simulink model "lab5_Sim"  (R2017b)
settings: Solver=VariableStepAuto  StartTime=0.0  StopTime=10.0  RelTol=1e-3
InitFcn:
  | load speech_signal
  | Fs= 8000;
  | Ts= 1/Fs;
  | 
  | DPRAM1_size = 2048;
  | DPRAM1_address_size = log2(DPRAM1_size);
  | 
  | FFT_size = 1024;
  | FFT_size_half = FFT_size;
  | FFT_frame_shift = 256;
  | FFT_frame_shift_Nbits = log2(FFT_frame_shift);
  | 
  | SysRate_Upsample_Factor = 32;
libraries: hdlsllib x16, simulink x5, dspxfrm3 x2, dspsigops x1
settings Model: Creator=Ross_admin  LastModifiedBy=h92j874
settings OptimizationCC: BlockReduction=off  ConditionallyExecuteInputs=off  DefaultParameterBehavior=Inlined
settings DebuggingCC: AlgebraicLoopMsg=error
settings HardwareCC: ProdBitPerPointer=32  ProdBitPerSizeT=32  ProdBitPerPtrDiffT=32  ProdLargestAtomicFloat=None  ProdIntDivRoundTo=Undefined  ProdEndianess=Unspecified  ProdWordSize=32  ProdHWDeviceType=ASIC/FPGA->ASIC/FPGA  TargetBitPerPointer=64  TargetBitPerSizeT=64  TargetBitPerPtrDiffT=64  TargetLongLongMode=on  TargetIntDivRoundTo=Zero  TargetEndianess=LittleEndian  TargetWordSize=64  TargetHWDeviceType=Custom Processor->MATLAB Host Computer  ProdEqTarget=off
settings CodeAppCC: StateflowObjectComments=on

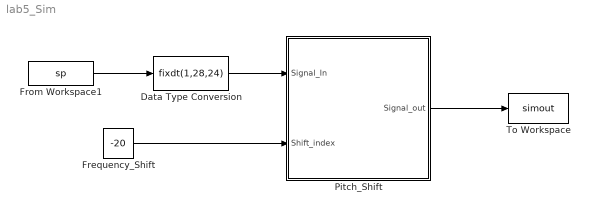
== system lab5_Sim ==
  Data Type Conversion : DataTypeConversion  OutDataTypeStr=fixdt(1,28,24)
  Frequency_Shift : Constant  Value=-20  OutDataTypeStr=int16
  From Workspace1 : FromWorkspace  VariableName=sp  SampleTime=0
  Pitch_Shift : Subsystem
  To Workspace : ToWorkspace  VariableName=simout  SampleTime=-1
  wires:
  Frequency_Shift/1 -> Pitch_Shift/2(Shift_index)
  Data Type Conversion/1 -> Pitch_Shift/1(Signal_In)
  From Workspace1/1 -> Data Type Conversion/1
  Pitch_Shift/1(Signal_out) -> To Workspace/1

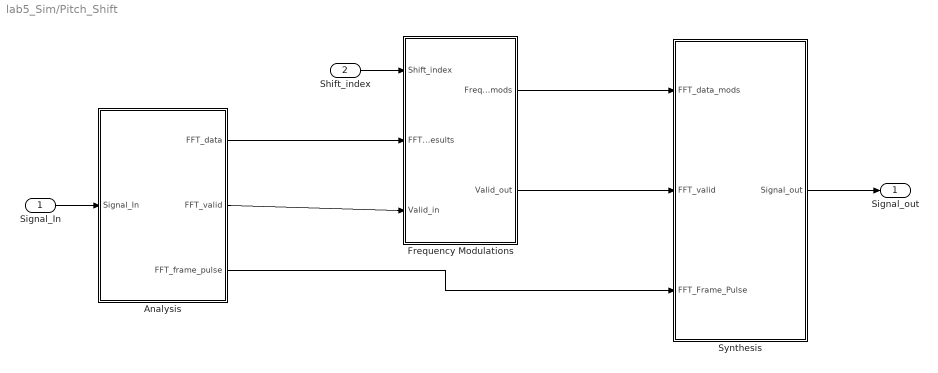
== system lab5_Sim/Pitch_Shift ==
  Signal_In : Inport
  Shift_index : Inport  Port=2
  Analysis : Subsystem
  Frequency Modulations : Subsystem
  Synthesis : Subsystem
  Signal_out : Outport
  wires:
  Signal_In/1 -> Analysis/1("Signal_In ")
  Analysis/1(FFT_data) -> Frequency Modulations/2(FFT_Results)
  Analysis/2(FFT_valid) -> Frequency Modulations/3(Valid_in)
  Shift_index/1 -> Frequency Modulations/1(Shift_index)
  Frequency Modulations/1(Frequency_mods) -> Synthesis/1(FFT_data_mods)
  Frequency Modulations/2(Valid_out) -> Synthesis/2(FFT_valid)
  Synthesis/1(Signal_out) -> Signal_out/1
  Analysis/3(FFT_frame_pulse) -> Synthesis/3(FFT_Frame_Pulse)

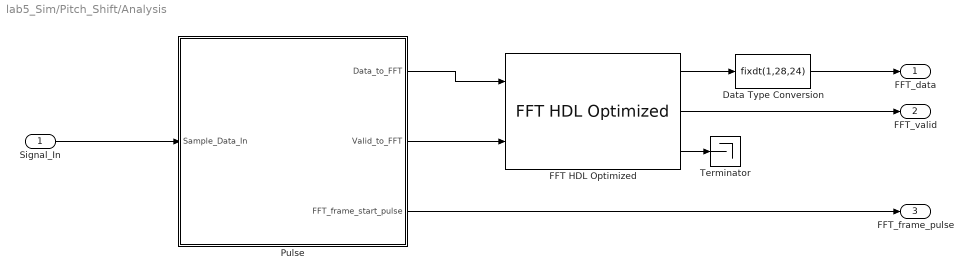
== system lab5_Sim/Pitch_Shift/Analysis ==
  "Signal_In " : Inport
  Data Type Conversion : DataTypeConversion  OutDataTypeStr=fixdt(1,28,24)
  FFT HDL Optimized : dspxfrm3/FFT HDL Optimized  FFTLength=1024  Architecture=Burst Radix 2  ComplexMultiplication=Use 4 multipliers and 2 adders  BitReversedOutput=off  BitReversedInput=off  Normalize=on  SimulateUsing=Code generation  RoundingMethod=Floor  ResetInputPort=off  StartOutputPort=off  EndOutputPort=off
      settings: SourceProductName=DSP System Toolbox  SourceProductBaseCode=DS
  "Pulse " : Subsystem
  Terminator : Terminator
  FFT_data : Outport
  FFT_valid : Outport  Port=2
  FFT_frame_pulse : Outport  Port=3
  wires:
  "Signal_In "/1 -> "Pulse "/1(Sample_Data_In)
  "Pulse "/3(FFT_frame_start_pulse) -> FFT_frame_pulse/1
  "Pulse "/2(Valid_to_FFT) -> FFT HDL Optimized/2
  FFT HDL Optimized/1 -> Data Type Conversion/1
  Data Type Conversion/1 -> FFT_data/1
  FFT HDL Optimized/2 -> FFT_valid/1
  FFT HDL Optimized/3 -> Terminator/1
  "Pulse "/1("Data_to_FFT ") -> FFT HDL Optimized/1

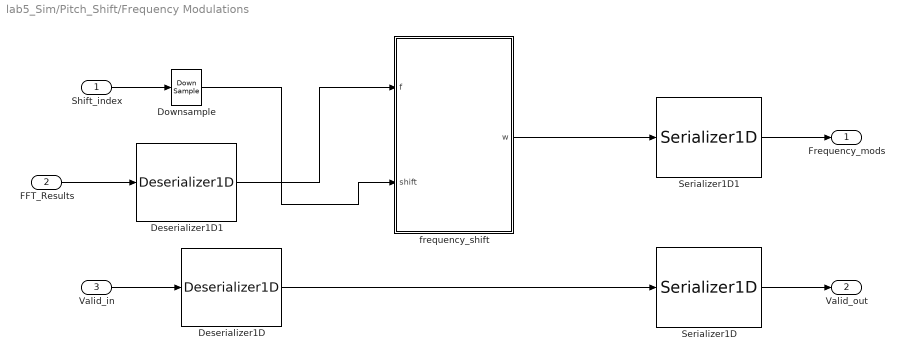
== system lab5_Sim/Pitch_Shift/Frequency Modulations ==
  Shift_index : Inport
  FFT_Results : Inport  Port=2
  Valid_in : Inport  Port=3
  Deserializer1D : hdlsllib/HDL Operations/Deserializer1D  Ratio=1024  IdleCycles=0  InitialCondition=0  startIn=off  validIn=off  validOut=off  inputDataDimensions=-1  inputSampleTime=-1  inputSignalType=auto
      settings: SourceProductName=HDL Coder  SourceProductBaseCode=HD
  Deserializer1D1 : hdlsllib/HDL Operations/Deserializer1D  Ratio=1024  IdleCycles=0  InitialCondition=0  startIn=off  validIn=off  validOut=off  inputDataDimensions=-1  inputSampleTime=-1  inputSignalType=auto
      settings: SourceProductName=HDL Coder  SourceProductBaseCode=HD
  Downsample : DownSample  N=FFT_size  RateOptions=Allow multirate processing
  Serializer1D : hdlsllib/HDL Operations/Serializer1D  Ratio=1024  IdleCycles=0  validIn=off  startOut=off  validOut=off  inputDataDimensions=-1  inputSampleTime=-1  inputSignalType=auto
      settings: SourceProductName=HDL Coder  SourceProductBaseCode=HD
  Serializer1D1 : hdlsllib/HDL Operations/Serializer1D  Ratio=1024  IdleCycles=0  validIn=off  startOut=off  validOut=off  inputDataDimensions=-1  inputSampleTime=-1  inputSignalType=auto
      settings: SourceProductName=HDL Coder  SourceProductBaseCode=HD
  "frequency_shift " : MATLAB Function  TreatAsAtomicUnit=on
  Frequency_mods : Outport
  Valid_out : Outport  Port=2
  wires:
  Serializer1D1/1 -> Frequency_mods/1
  FFT_Results/1 -> Deserializer1D1/1
  Valid_in/1 -> Deserializer1D/1
  Shift_index/1 -> Downsample/1
  "frequency_shift "/1(w) -> Serializer1D1/1
  Serializer1D/1 -> Valid_out/1
  Downsample/1 -> "frequency_shift "/2(shift)
  Deserializer1D1/1 -> "frequency_shift "/1(f)
  Deserializer1D/1 -> Serializer1D/1

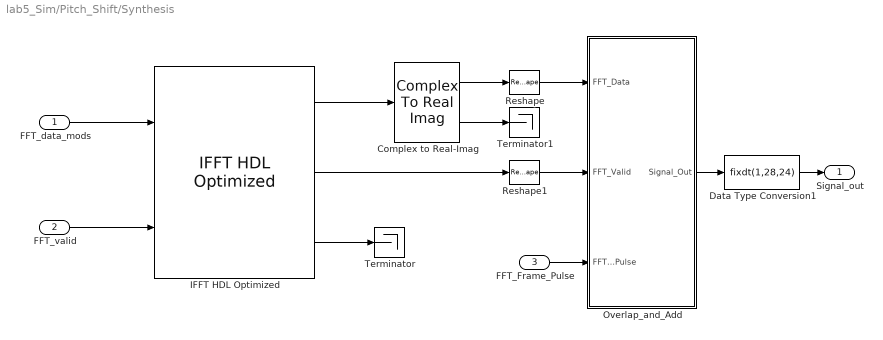
== system lab5_Sim/Pitch_Shift/Synthesis ==
  FFT_data_mods : Inport
  FFT_valid : Inport  Port=2
  FFT_Frame_Pulse : Inport  Port=3
  Complex to Real-Imag : ComplexToRealImag
  Data Type Conversion1 : DataTypeConversion  OutDataTypeStr=fixdt(1,28,24)
  IFFT HDL Optimized : dspxfrm3/IFFT HDL Optimized  FFTLength=1024  Architecture=Burst Radix 2  ComplexMultiplication=Use 4 multipliers and 2 adders  BitReversedOutput=off  BitReversedInput=off  Normalize=on  SimulateUsing=Code generation  RoundingMethod=Floor  ResetInputPort=off  StartOutputPort=off  EndOutputPort=off
      settings: SourceProductName=DSP System Toolbox  SourceProductBaseCode=DS
  Overlap_and_Add : Subsystem
  Reshape : Reshape
  Reshape1 : Reshape
  Terminator : Terminator
  Terminator1 : Terminator
  Signal_out : Outport
  wires:
  FFT_data_mods/1 -> IFFT HDL Optimized/1
  FFT_valid/1 -> IFFT HDL Optimized/2
  IFFT HDL Optimized/3 -> Terminator/1
  IFFT HDL Optimized/1 -> Complex to Real-Imag/1
  Complex to Real-Imag/1 -> Reshape/1
  Complex to Real-Imag/2 -> Terminator1/1
  IFFT HDL Optimized/2 -> Reshape1/1
  Reshape1/1 -> Overlap_and_Add/2(FFT_Valid)
  Reshape/1 -> Overlap_and_Add/1(FFT_Data)
  FFT_Frame_Pulse/1 -> Overlap_and_Add/3(FFT_Frame_Pulse)
  Data Type Conversion1/1 -> Signal_out/1
  Overlap_and_Add/1(Signal_Out) -> Data Type Conversion1/1

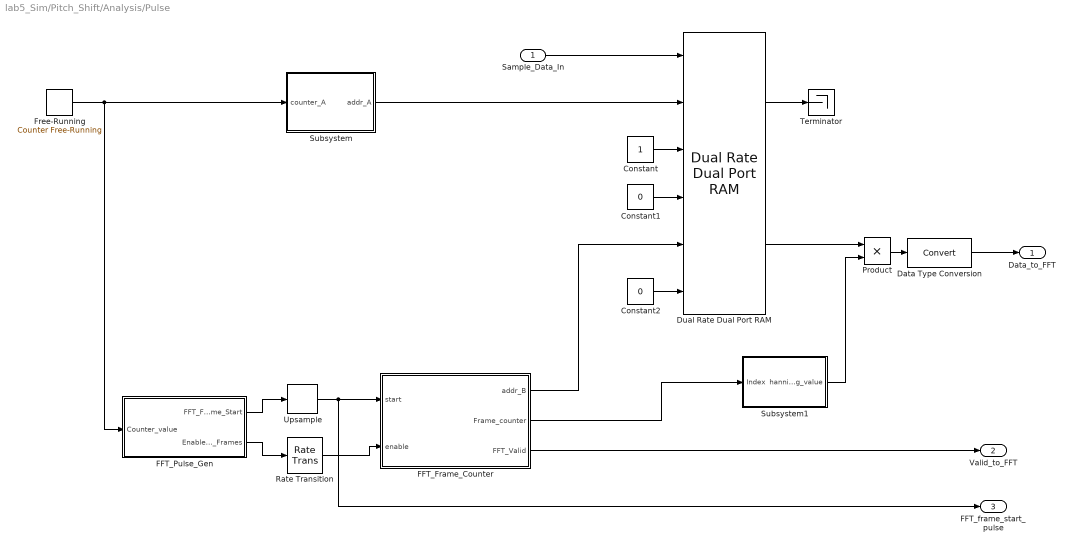
== system lab5_Sim/Pitch_Shift/Analysis/Pulse  ==
  Sample_Data_In : Inport
  Constant : Constant  OutDataTypeStr=boolean
  Constant1 : Constant  Value=0  OutDataTypeStr=fixdt(1,28,24)
  Constant2 : Constant  Value=0  OutDataTypeStr=boolean
  Data Type Conversion : DataTypeConversion
  Dual Rate Dual Port RAM : hdlsllib/HDL RAMs/Dual Rate Dual Port RAM  ram_size=DPRAM1_address_size
      settings: SourceProductName=HDL Coder  SourceProductBaseCode=HD
  FFT_Frame_Counter : Subsystem
  FFT_Pulse_Gen : Subsystem
  Free-Running : simulink/Sources/Counter Free-Running  NumBits=DPRAM1_address_size  tsamp=Ts
  Product : Product
  Rate Transition : RateTransition
  Subsystem : Subsystem
  Subsystem1 : Subsystem
  Terminator : Terminator
  Upsample : dspsigops/Upsample  N=SysRate_Upsample_Factor  phase=0  RateOptions=Allow multirate processing  ic=0  mode=Unused parameter value
  "Data_to_FFT " : Outport
  Valid_to_FFT : Outport  Port=2
  FFT_frame_start_pulse : Outport  Port=3
  wires:
  FFT_Pulse_Gen/2(Enable_FFT_Frames) -> Rate Transition/1
  Subsystem1/1(hanning_value) -> Product/2
  Subsystem/1(addr_A) -> Dual Rate Dual Port RAM/2
  FFT_Frame_Counter/1(addr_B) -> Dual Rate Dual Port RAM/5
  Dual Rate Dual Port RAM/2 -> Product/1
  FFT_Frame_Counter/3("FFT_Valid ") -> Valid_to_FFT/1
  Upsample/1 -> FFT_frame_start_pulse/1, FFT_Frame_Counter/1("start ")
  Rate Transition/1 -> FFT_Frame_Counter/2("enable ")
  FFT_Frame_Counter/2("Frame_counter ") -> Subsystem1/1(Index)
  FFT_Pulse_Gen/1("FFT_Frame_Start ") -> Upsample/1
  Free-Running/1 -> Subsystem/1("counter_A "), FFT_Pulse_Gen/1("Counter_value ")
  Constant2/1 -> Dual Rate Dual Port RAM/6
  Constant/1 -> Dual Rate Dual Port RAM/3
  Sample_Data_In/1 -> Dual Rate Dual Port RAM/1
  Constant1/1 -> Dual Rate Dual Port RAM/4
  Product/1 -> Data Type Conversion/1
  Data Type Conversion/1 -> "Data_to_FFT "/1
  Dual Rate Dual Port RAM/1 -> Terminator/1

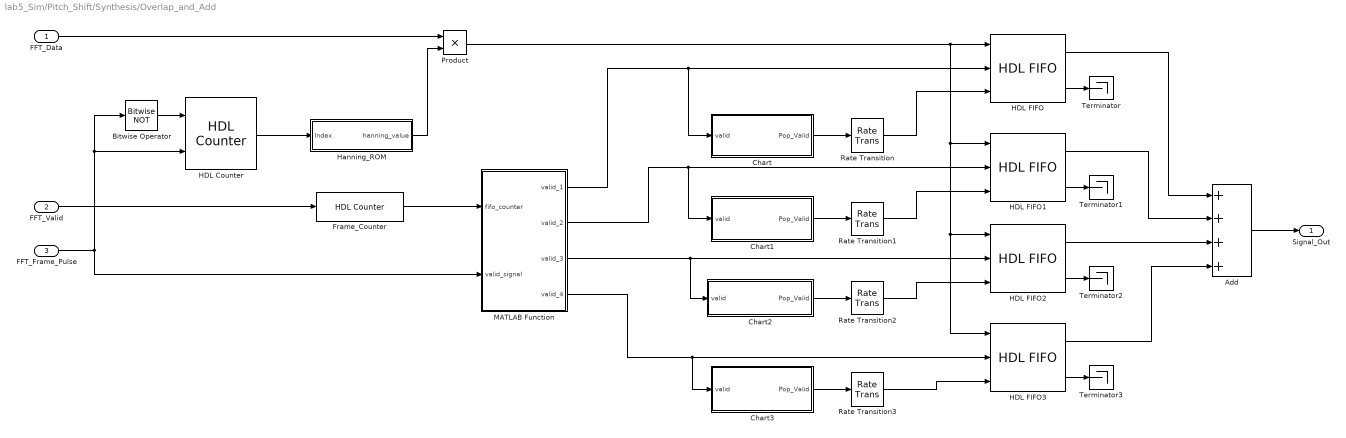
== system lab5_Sim/Pitch_Shift/Synthesis/Overlap_and_Add ==
  FFT_Data : Inport
  FFT_Valid : Inport  Port=2
  FFT_Frame_Pulse : Inport  Port=3
  Add : Sum  Inputs=4
  Bitwise Operator : simulink/Logic and Bit Operations/Bitwise Operator  logicop=NOT  UseBitMask=off  BitMask=bin2dec('11011001')  BitMaskRealWorld=Stored Integer
  Chart : Stateflow chart  TreatAsAtomicUnit=on
  Chart1 : Stateflow chart  TreatAsAtomicUnit=on
  Chart2 : Stateflow chart  TreatAsAtomicUnit=on
  Chart3 : Stateflow chart  TreatAsAtomicUnit=on
  Frame_Counter : hdlsllib/Sources/HDL Counter  CountType=Free running  CountInit=2  CountStep=1  CountMax=3  CountFromType=Initial value  CountFrom=2  CountResetPort=off  CountLoadPort=off  CountEnbPort=on  CountDirPort=off  CountDataType=Unsigned  CountWordLen=2  CountFracLen=0  CountSampTime=1
      settings: SourceProductBaseCode=HD
  HDL Counter : hdlsllib/Sources/HDL Counter  CountType=Count limited  CountInit=0  CountStep=1  CountMax=FFT_size  CountFromType=Initial value  CountFrom=0  CountResetPort=on  CountLoadPort=off  CountEnbPort=on  CountDirPort=off  CountDataType=Unsigned  CountWordLen=DPRAM1_address_size  CountFracLen=0  CountSampTime=1
      settings: SourceProductBaseCode=HD
  HDL FIFO{,1..3} (4 alike) : hdlsllib/HDL RAMs/HDL FIFO  fifo_size=FFT_size  ratio=SysRate_Upsample_Factor  push_msg=Warning  pop_msg=Warning  show_empty=off  show_full=on  show_num=off
      settings: SourceProductName=HDL Coder  SourceProductBaseCode=HD
  Hanning_ROM : Subsystem
  MATLAB Function : MATLAB Function  TreatAsAtomicUnit=on
  Product : Product
  Rate Transition{,1..3} (4 alike) : RateTransition  OutPortSampleTimeOpt=Multiple of input port sample time  OutPortSampleTimeMultiple=SysRate_Upsample_Factor  OutPortSampleTime=SysRate_Upsample_Factor
  Terminator{,1..3} (4 alike) : Terminator
  Signal_Out : Outport
  wires:
  Bitwise Operator/1 -> HDL Counter/1
  FFT_Frame_Pulse/1 -> MATLAB Function/2(valid_signal), HDL Counter/2, Bitwise Operator/1
  FFT_Data/1 -> Product/1
  HDL Counter/1 -> Hanning_ROM/1(Index)
  Hanning_ROM/1(hanning_value) -> Product/2
  FFT_Valid/1 -> Frame_Counter/1
  Frame_Counter/1 -> MATLAB Function/1(fifo_counter)
  Chart3/1(Pop_Valid) -> Rate Transition3/1
  Add/1 -> Signal_Out/1
  Product/1 -> HDL FIFO1/1, HDL FIFO3/1, HDL FIFO2/1, HDL FIFO/1
  MATLAB Function/2(valid_2) -> Chart1/1(valid), HDL FIFO1/2
  MATLAB Function/3(valid_3) -> Chart2/1(valid), HDL FIFO2/2
  MATLAB Function/4(valid_4) -> Chart3/1(valid), HDL FIFO3/2
  MATLAB Function/1(valid_1) -> Chart/1(valid), HDL FIFO/2
  Rate Transition3/1 -> HDL FIFO3/3
  Rate Transition2/1 -> HDL FIFO2/3
  Rate Transition1/1 -> HDL FIFO1/3
  Rate Transition/1 -> HDL FIFO/3
  HDL FIFO/1 -> Add/1
  HDL FIFO1/1 -> Add/2
  HDL FIFO2/1 -> Add/3
  HDL FIFO3/1 -> Add/4
  HDL FIFO1/2 -> Terminator1/1
  HDL FIFO2/2 -> Terminator2/1
  HDL FIFO3/2 -> Terminator3/1
  HDL FIFO/2 -> Terminator/1
  Chart1/1(Pop_Valid) -> Rate Transition1/1
  Chart/1(Pop_Valid) -> Rate Transition/1
  Chart2/1(Pop_Valid) -> Rate Transition2/1

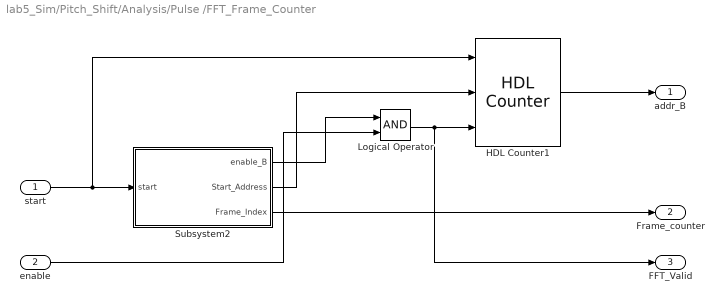
== system lab5_Sim/Pitch_Shift/Analysis/Pulse /FFT_Frame_Counter ==
  "start " : Inport
  "enable " : Inport  Port=2
  HDL Counter1 : hdlsllib/Sources/HDL Counter  CountType=Count limited  CountInit=DPRAM1_size-10  CountStep=1  CountMax=1024  CountFromType=Specify  CountFrom=DPRAM1_size-10  CountResetPort=off  CountLoadPort=on  CountEnbPort=on  CountDirPort=off  CountDataType=Unsigned  CountWordLen=DPRAM1_address_size  CountFracLen=0  CountSampTime=1
      settings: SourceProductBaseCode=HD
  Logical Operator : Logic  AllPortsSameDT=off  OutDataTypeStr=boolean
  Subsystem2 : Subsystem
  addr_B : Outport
  "Frame_counter " : Outport  Port=2
  "FFT_Valid " : Outport  Port=3
  wires:
  Subsystem2/1(enable_B) -> Logical Operator/1
  "start "/1 -> HDL Counter1/1, Subsystem2/1("start ")
  HDL Counter1/1 -> addr_B/1
  Logical Operator/1 -> "FFT_Valid "/1, HDL Counter1/3
  Subsystem2/2(Start_Address) -> HDL Counter1/2
  Subsystem2/3("Frame_Index ") -> "Frame_counter "/1
  "enable "/1 -> Logical Operator/2

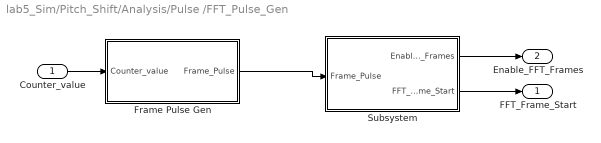
== system lab5_Sim/Pitch_Shift/Analysis/Pulse /FFT_Pulse_Gen ==
  "Counter_value " : Inport
  "Frame Pulse Gen " : Subsystem
  Subsystem : Subsystem
  "FFT_Frame_Start " : Outport
  Enable_FFT_Frames : Outport  Port=2
  wires:
  "Frame Pulse Gen "/1("Frame_Pulse ") -> Subsystem/1("Frame_Pulse ")
  Subsystem/1(Enable_FFT_Frames) -> Enable_FFT_Frames/1
  Subsystem/2("FFT_Frame_Start ") -> "FFT_Frame_Start "/1
  "Counter_value "/1 -> "Frame Pulse Gen "/1("Counter_value ")

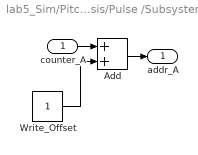
== system lab5_Sim/Pitch_Shift/Analysis/Pulse /Subsystem ==
  "counter_A " : Inport
  Add : Sum  AccumDataTypeStr=fixdt(0,11,0)
  "Write_Offset " : Constant  OutDataTypeStr=fixdt(0,11,0)
  addr_A : Outport
  wires:
  "Write_Offset "/1 -> Add/2
  "counter_A "/1 -> Add/1
  Add/1 -> addr_A/1

== system lab5_Sim/Pitch_Shift/Analysis/Pulse /Subsystem1 ==
  Index : Inport
  1-D Lookup Table1 : Lookup_n-D  NumberOfTableDimensions=1  LookupTableObject=''  BreakpointsForDimension1=[0:FFT_size]  BreakpointsForDimension1FirstPoint=10  BreakpointsForDimension2FirstPoint=10  BreakpointsForDimension1Spacing=12  BreakpointsForDimension2Spacing=12  IndexSearchMethod=Evenly spaced points  Table=hanning(FFT_size+1)  InterpMethod=Flat  DiagnosticForOutOfRangeInput=Error  OutDataTypeStr=fixdt(1,16,14)  RndMeth=Simplest  InputSameDT=on
  Unit Delay : UnitDelay  SampleTime=-1
  hanning_value : Outport
  wires:
  1-D Lookup Table1/1 -> Unit Delay/1
  Unit Delay/1 -> hanning_value/1
  Index/1 -> 1-D Lookup Table1/1

== system lab5_Sim/Pitch_Shift/Synthesis/Overlap_and_Add/Hanning_ROM ==
  Index : Inport
  1-D Lookup Table : Lookup_n-D  NumberOfTableDimensions=1  LookupTableObject=''  BreakpointsForDimension1=[0:FFT_size]  BreakpointsForDimension1FirstPoint=10  BreakpointsForDimension2FirstPoint=10  BreakpointsForDimension1Spacing=12  BreakpointsForDimension2Spacing=12  IndexSearchMethod=Evenly spaced points  Table=hanning(FFT_size+1)  InterpMethod=Flat  DiagnosticForOutOfRangeInput=Error  OutDataTypeStr=fixdt(1,16,14)  RndMeth=Simplest  InputSameDT=on
  Unit Delay : UnitDelay  SampleTime=-1
  hanning_value : Outport
  wires:
  Unit Delay/1 -> hanning_value/1
  Index/1 -> 1-D Lookup Table/1
  1-D Lookup Table/1 -> Unit Delay/1

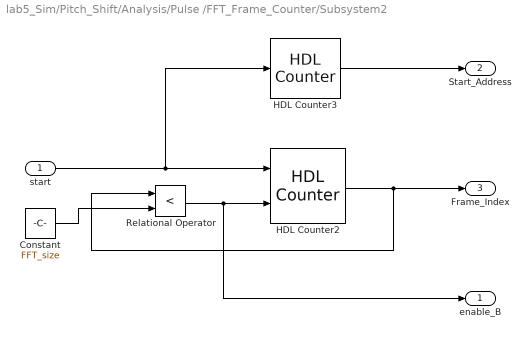
== system lab5_Sim/Pitch_Shift/Analysis/Pulse /FFT_Frame_Counter/Subsystem2 ==
  "start " : Inport
  Constant : Constant  Value=FFT_size
  HDL Counter2 : hdlsllib/Sources/HDL Counter  CountType=Count limited  CountInit=0  CountStep=1  CountMax=FFT_size  CountFromType=Specify  CountFrom=0  CountResetPort=on  CountLoadPort=off  CountEnbPort=on  CountDirPort=off  CountDataType=Unsigned  CountWordLen=DPRAM1_address_size  CountFracLen=0  CountSampTime=1
      settings: SourceProductBaseCode=HD
  HDL Counter3 : hdlsllib/Sources/HDL Counter  CountType=Free running  CountInit=0  CountStep=FFT_frame_shift  CountMax=DPRAM1_size  CountFromType=Specify  CountFrom=0  CountResetPort=off  CountLoadPort=off  CountEnbPort=on  CountDirPort=off  CountDataType=Unsigned  CountWordLen=DPRAM1_address_size  CountFracLen=0  CountSampTime=1
      settings: SourceProductBaseCode=HD
  Relational Operator : RelationalOperator  Operator=<  OutDataTypeStr=boolean  RndMeth=Nearest
  enable_B : Outport
  Start_Address : Outport  Port=2
  "Frame_Index " : Outport  Port=3
  wires:
  HDL Counter2/1 -> Relational Operator/1, "Frame_Index "/1
  HDL Counter3/1 -> Start_Address/1
  "start "/1 -> HDL Counter2/1, HDL Counter3/1
  Relational Operator/1 -> enable_B/1, HDL Counter2/2
  Constant/1 -> Relational Operator/2

== system lab5_Sim/Pitch_Shift/Analysis/Pulse /FFT_Pulse_Gen/Frame Pulse Gen  ==
  "Counter_value " : Inport
  Bit Slice : hdlsllib/Logic and Bit Operations/Bit Slice  lidx=7  ridx=0
  Compare To Zero : simulink/Logic and Bit Operations/Compare To Zero  relop===  OutDataTypeStr=boolean
  "Frame_Pulse " : Outport
  wires:
  Compare To Zero/1 -> "Frame_Pulse "/1
  Bit Slice/1 -> Compare To Zero/1
  "Counter_value "/1 -> Bit Slice/1

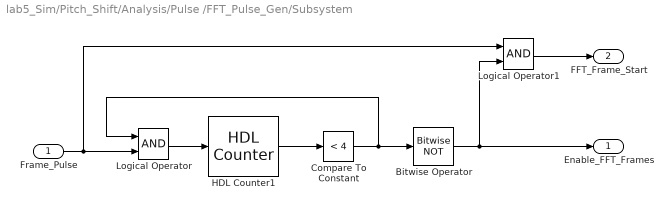
== system lab5_Sim/Pitch_Shift/Analysis/Pulse /FFT_Pulse_Gen/Subsystem ==
  "Frame_Pulse " : Inport
  Bitwise Operator : simulink/Logic and Bit Operations/Bitwise Operator  logicop=NOT  UseBitMask=off  BitMask=bin2dec('11011001')  BitMaskRealWorld=Stored Integer
  Compare To Constant : simulink/Logic and Bit Operations/Compare To Constant  relop=<  const=4  OutDataTypeStr=boolean
  HDL Counter1 : hdlsllib/Sources/HDL Counter  CountType=Count limited  CountInit=0  CountStep=1  CountMax=4  CountFromType=Specify  CountFrom=0  CountResetPort=off  CountLoadPort=off  CountEnbPort=on  CountDirPort=off  CountDataType=Unsigned  CountWordLen=5  CountFracLen=0  CountSampTime=1
      settings: SourceProductBaseCode=HD
  Logical Operator : Logic  AllPortsSameDT=off  OutDataTypeStr=boolean
  Logical Operator1 : Logic  AllPortsSameDT=off  OutDataTypeStr=boolean
  Enable_FFT_Frames : Outport
  "FFT_Frame_Start " : Outport  Port=2
  wires:
  Logical Operator/1 -> HDL Counter1/1
  HDL Counter1/1 -> Compare To Constant/1
  Compare To Constant/1 -> Logical Operator/1, Bitwise Operator/1
  "Frame_Pulse "/1 -> Logical Operator1/1, Logical Operator/2
  Logical Operator1/1 -> "FFT_Frame_Start "/1
  Bitwise Operator/1 -> Enable_FFT_Frames/1, Logical Operator1/2

== matlab function lab5_Sim/Pitch_Shift/Synthesis/Overlap_and_Add/MATLAB Function ==
  data: fifo_counter input; valid_1 output; valid_signal input; valid_2 output; valid_3 output; valid_4 output
function [valid_1,valid_2,valid_3,valid_4] = fcn(fifo_counter,valid_signal)
%#codegen

switch fifo_counter
    case 0
        valid_1 = valid_signal;
        valid_2 = false;
        valid_3 = false;
        valid_4 = false;
    case 1
        valid_1 = false;
        valid_2 = valid_signal;
        valid_3 = false;
        valid_4 = false;
    case 2
        valid_1 = false;
        valid_2 = false;
        valid_3 = valid_signal;
        valid_4 = false;
    case 3
        valid_1 = false;
        valid_2 = false;
        valid_3 = false;
        valid_4 = valid_signal;
    otherwise
        valid_1 = false;
        valid_2 = false;
        valid_3 = false;
        valid_4 = false;
end

== matlab function lab5_Sim/Pitch_Shift/Frequency Modulations/frequency_shift  ==
  data: f input; shift input; w output
function w = fcn(f,shift)

N = length(f);
w = complex(zeros(N,1));

if shift == 0
    w = f;
else
    
    zf = f(1);            % dc term
    pf = f(2:N/2);        % positive frequencies
    lf = f(N/2 + 1);      % last positive frequency
    nf = f(N/2 + 2:N);  % negative frequencies (paired with positive frequencies)
    
    w(1) = zf;
    w(N/2+1) = complex(0);                   % just zero frequency at -pi since both positive and negative frequencies map here when shifted
        
    if shift > 0  % increase the frequencies
        
        for i=1:shift
            w(i) = complex(0);                   % fill in vacated positive frequencies with zeros
        end
        w(shift+1:N/2) = pf(1:end-shift+1);      % shift positive frequencies to the right

        w(N/2+2:end-shift) = nf(shift + 1:end);  % shift negative frequencies to the left
        for i=N-shift+1:N
            w(i) = complex(0);                   % fill in vacated negative frequencies with zeros
        end
        
    end
    if shift < 0  % decrease the frequencies
      
        nshift = abs(shift);
        
        w(2:N/2-nshift) = pf(nshift+1:end);      % shift positive frequencies to the left
        for i=N/2-nshift+2:N/2+1
            w(i) = complex(0);                   % fill in vacated positive frequencies with zeros
        end
        
        w(N/2+2+nshift:N) = nf(1:end-nshift);      % shift negative frequencies to the right
        for i=N/2+2:N/2+2+nshift-1
            w(i) = complex(0);                   % fill in vacated negative frequencies with zeros
        end
        


    end
end

== stateflow chart lab5_Sim/Pitch_Shift/Synthesis/Overlap_and_Add/Chart ==
  state Start_up
    entry: Pop_Valid=fi(0,0,1,0);
  state valid_low
    entry:Pop_Valid=fi(0,0,1,0);
  state valid_high
    entry:Pop_Valid=fi(0,0,1,0);
  state Pop_assert
    entry:Pop_Valid=fi(1,0,1,0);
  (default) -> Start_up
  Start_up -> valid_low : [valid==0]
  valid_high -> Pop_assert [order 1] : [valid==0]
  valid_low -> valid_high [order 1] : [valid==1]
  valid_low -> valid_low [order 2] : [valid==0]
  valid_high -> valid_high [order 2] : [valid==1]
  data: valid input; Pop_Valid output

== stateflow chart lab5_Sim/Pitch_Shift/Synthesis/Overlap_and_Add/Chart1 ==
  state Start_up
    entry: Pop_Valid=fi(0,0,1,0);
  state valid_low
    entry:Pop_Valid=fi(0,0,1,0);
  state valid_high
    entry:Pop_Valid=fi(0,0,1,0);
  state Pop_assert
    entry:Pop_Valid=fi(1,0,1,0);
  (default) -> Start_up
  Start_up -> valid_low : [valid==0]
  valid_high -> Pop_assert [order 1] : [valid==0]
  valid_low -> valid_high [order 1] : [valid==1]
  valid_low -> valid_low [order 2] : [valid==0]
  valid_high -> valid_high [order 2] : [valid==1]
  data: valid input; Pop_Valid output

== stateflow chart lab5_Sim/Pitch_Shift/Synthesis/Overlap_and_Add/Chart2 ==
  state Start_up
    entry: Pop_Valid=fi(0,0,1,0);
  state valid_low
    entry:Pop_Valid=fi(0,0,1,0);
  state valid_high
    entry:Pop_Valid=fi(0,0,1,0);
  state Pop_assert
    entry:Pop_Valid=fi(1,0,1,0);
  (default) -> Start_up
  Start_up -> valid_low : [valid==0]
  valid_high -> Pop_assert [order 1] : [valid==0]
  valid_low -> valid_high [order 1] : [valid==1]
  valid_low -> valid_low [order 2] : [valid==0]
  valid_high -> valid_high [order 2] : [valid==1]
  data: valid input; Pop_Valid output

== stateflow chart lab5_Sim/Pitch_Shift/Synthesis/Overlap_and_Add/Chart3 ==
  state Start_up
    entry: Pop_Valid=fi(0,0,1,0);
  state valid_low
    entry:Pop_Valid=fi(0,0,1,0);
  state valid_high
    entry:Pop_Valid=fi(0,0,1,0);
  state Pop_assert
    entry:Pop_Valid=fi(1,0,1,0);
  (default) -> Start_up
  Start_up -> valid_low : [valid==0]
  valid_low -> valid_high [order 1] : [valid==1]
  valid_high -> Pop_assert [order 1] : [valid==0]
  valid_low -> valid_low [order 2] : [valid==0]
  valid_high -> valid_high [order 2] : [valid==1]
  data: valid input; Pop_Valid output
